simulink model "lyapunov11"  (R2015a)
settings: Solver=ode4  StartTime=0.0  StopTime=15  FixedStep=0.001  RelTol=1e-3
values from neighbouring files (symbols this model uses):
  a = 0.15    [RunLyapunov11.m]    (also in lyapunovInit.m = 0.13)
  kpsi = 10    [RunLyapunov11.m]    (also in lyapunovInit.m)
  kx = 10    [RunLyapunov11.m]    (also in lyapunovInit.m = 25)
  ky = 10    [RunLyapunov11.m]    (also in lyapunovInit.m = 25)
  r = 0.1    [RunLyapunov11.m]    (also in lyapunovInit.m)
  R = 2    [RunLyapunov11.m]    (also in lyapunovInit.m)
  theta0 = pi    (= 3.14159265359)    [RunLyapunov11.m]    (also in lyapunovInit.m)
  wd = 0.5    [RunLyapunov11.m]    (also in lyapunovInit.m)
  x0 = 2.3    [RunLyapunov11.m]    (also in lyapunovInit.m)
  y0 = 0    [RunLyapunov11.m]    (also in lyapunovInit.m)
undefined symbols (not defined in the file or in its folder): lyapu
settings Model: CovModelRefEnable=off  Creator=Subodh  LastModifiedBy=smishra
settings DataIOCC: LimitDataPoints=off  SaveFormat=Dataset
settings HardwareCC: ProdBitPerPointer=64  ProdLargestAtomicFloat=Float  ProdIntDivRoundTo=Zero  ProdEndianess=LittleEndian  ProdHWDeviceType=Specified
settings GRTTargetCC: GeneratePreprocessorConditionals=Use local settings

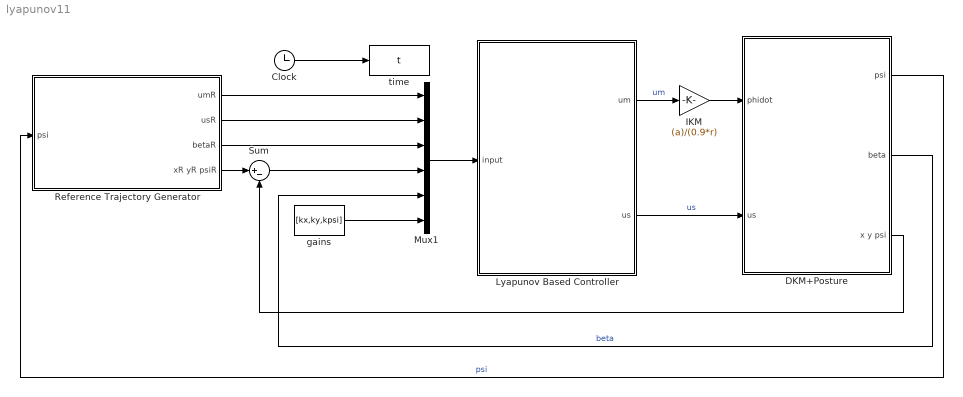
== system lyapunov11 ==
  Clock : Clock
  DKM+Posture : Subsystem
  IKM : Gain  Gain=(a)/(0.9*r)
  Lyapunov Based Controller : Subsystem
  Mux1 : Mux  Inputs=6
  Reference Trajectory Generator : Subsystem
  Sum : Sum  Inputs=|+-
  gains : Constant  Value=[kx,ky,kpsi]
  time : ToWorkspace  VariableName=t  SampleTime=-1
  wires:
  Lyapunov Based Controller/2(us) -> DKM+Posture/2(us)  "us"
  Lyapunov Based Controller/1(um) -> IKM/1  "um"
  IKM/1 -> DKM+Posture/1(phidot)
  DKM+Posture/3(x y psi) -> Sum/2
  Clock/1 -> time/1
  Reference Trajectory Generator/1(umR) -> Mux1/1
  Reference Trajectory Generator/2(usR) -> Mux1/2
  Reference Trajectory Generator/3(betaR) -> Mux1/3
  Reference Trajectory Generator/4(xR yR psiR) -> Sum/1
  Sum/1 -> Mux1/4
  DKM+Posture/2(beta) -> Mux1/5  "beta"
  DKM+Posture/1(psi) -> Reference Trajectory Generator/1(psi)  "psi"
  Mux1/1 -> Lyapunov Based Controller/1(input)
  gains/1 -> Mux1/6

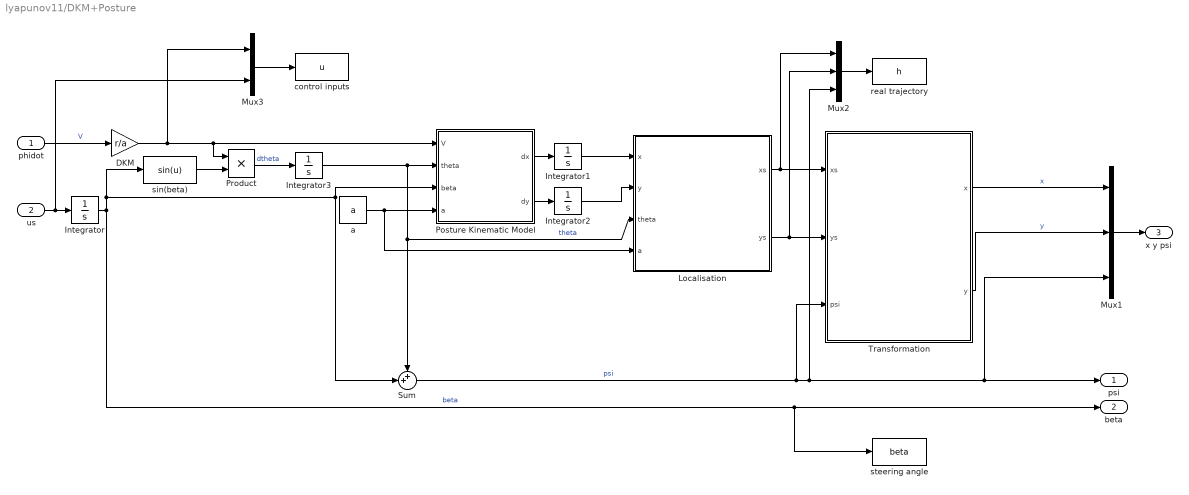
== system lyapunov11/DKM+Posture ==
  phidot : Inport
  us : Inport  Port=2
  DKM : Gain  Gain=r/a
  Integrator : Integrator
  Integrator1 : Integrator  InitialCondition=x0
  Integrator2 : Integrator  InitialCondition=y0
  Integrator3 : Integrator  InitialCondition=theta0
  Localisation : MATLAB Function  TreatAsAtomicUnit=on
  Mux1 : Mux  Inputs=3
  Mux2 : Mux  Inputs=3
  Mux3 : Mux  Inputs=2
  Posture Kinematic Model : MATLAB Function  TreatAsAtomicUnit=on
  Product : Product
  Sum : Sum  Inputs=++|
  Transformation : MATLAB Function  TreatAsAtomicUnit=on
  a : Constant  Value=a
  control inputs : ToWorkspace  VariableName=u  SampleTime=-1
  real trajectory : ToWorkspace  VariableName=h  SampleTime=-1
  sin(beta) : Fcn  Expr=sin(u)
  steering angle : ToWorkspace  VariableName=beta  SampleTime=-1
  psi : Outport
  beta : Outport  Port=2
  x y psi : Outport  Port=3
  wires:
  sin(beta)/1 -> Product/2
  us/1 -> Mux3/2, Integrator/1
  Product/1 -> Integrator3/1  "dtheta"
  Sum/1 -> Transformation/3(psi), Mux2/3, psi/1, Mux1/3  "psi"
  Integrator3/1 -> Sum/1, Localisation/3(theta), Posture Kinematic Model/2(theta)  "theta"
  Posture Kinematic Model/1(dx) -> Integrator1/1
  Posture Kinematic Model/2(dy) -> Integrator2/1
  Integrator/1 -> sin(beta)/1, Posture Kinematic Model/3(beta), Sum/2, steering angle/1, beta/1  "beta"
  Integrator2/1 -> Localisation/2(y)
  Localisation/2(ys) -> Mux2/2, Transformation/2(ys)
  DKM/1 -> Mux3/1, Product/1, Posture Kinematic Model/1(V)
  phidot/1 -> DKM/1  "V"
  Transformation/1(x) -> Mux1/1  "x"
  Transformation/2(y) -> Mux1/2  "y"
  Mux1/1 -> x y psi/1
  a/1 -> Localisation/4(a), Posture Kinematic Model/4(a)
  Integrator1/1 -> Localisation/1(x)
  Localisation/1(xs) -> Mux2/1, Transformation/1(xs)
  Mux2/1 -> real trajectory/1
  Mux3/1 -> control inputs/1

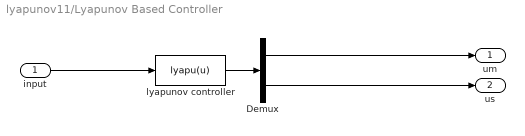
== system lyapunov11/Lyapunov Based Controller ==
  input : Inport
  Demux : Demux  Outputs=2
  lyapunov controller : MATLABFcn  MATLABFcn=lyapu(u)  OutputDimensions=2
  um : Outport
  us : Outport  Port=2
  wires:
  input/1 -> lyapunov controller/1
  Demux/2 -> us/1
  Demux/1 -> um/1
  lyapunov controller/1 -> Demux/1

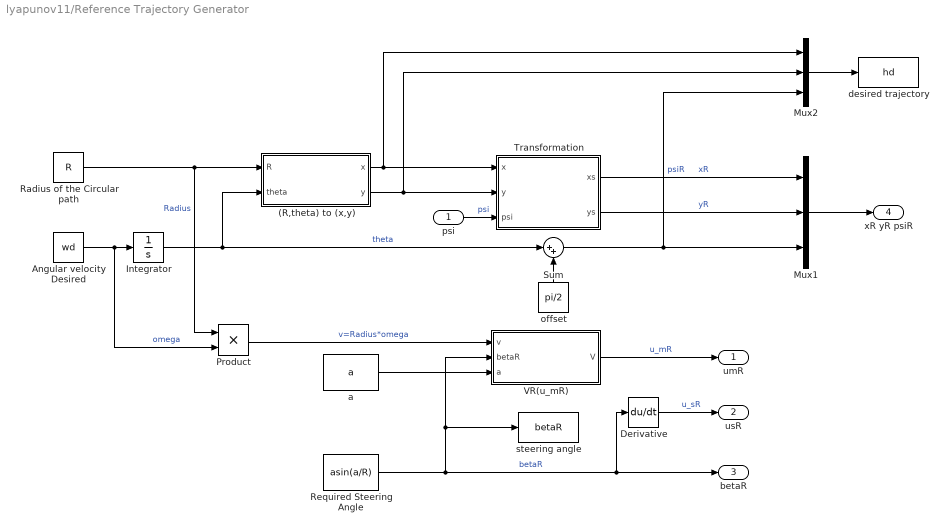
== system lyapunov11/Reference Trajectory Generator ==
  psi : Inport
  (R,theta) to (x,y) : MATLAB Function  TreatAsAtomicUnit=on
  Angular velocity Desired : Constant  Value=wd
  Derivative : Derivative
  Integrator : Integrator
  Mux1 : Mux  Inputs=3
  Mux2 : Mux  Inputs=3
  Product : Product
  Radius of the Circular path : Constant  Value=R
  Required Steering Angle : Constant  Value=asin(a/R)
  Sum : Sum  Inputs=|++
  Transformation : MATLAB Function  TreatAsAtomicUnit=on
  VR(u_mR) : MATLAB Function  TreatAsAtomicUnit=on
  a : Constant  Value=a
  desired trajectory : ToWorkspace  VariableName=hd  SampleTime=-1
  offset : Constant  Value=pi/2
  steering angle : ToWorkspace  VariableName=betaR  SampleTime=-1
  umR : Outport
  usR : Outport  Port=2
  betaR : Outport  Port=3
  xR yR psiR : Outport  Port=4
  wires:
  Radius of the Circular path/1 -> Product/1, (R,theta) to (x,y)/1(R)  "Radius"
  Angular velocity Desired/1 -> Product/2, Integrator/1  "omega"
  VR(u_mR)/1(V) -> umR/1  "u_mR"
  Required Steering Angle/1 -> Derivative/1, betaR/1, steering angle/1, VR(u_mR)/2(betaR)  "betaR"
  Derivative/1 -> usR/1  "u_sR"
  Product/1 -> VR(u_mR)/1(v)  "v=Radius*omega"
  psi/1 -> Transformation/3(psi)  "psi"
  Transformation/1(xs) -> Mux1/1  "xR"
  Transformation/2(ys) -> Mux1/2  "yR"
  (R,theta) to (x,y)/1(x) -> Mux2/1, Transformation/1(x)
  (R,theta) to (x,y)/2(y) -> Mux2/2, Transformation/2(y)
  offset/1 -> Sum/2
  Integrator/1 -> (R,theta) to (x,y)/2(theta), Sum/1  "theta"
  Mux1/1 -> xR yR psiR/1
  a/1 -> VR(u_mR)/3(a)
  Sum/1 -> Mux2/3, Mux1/3  "psiR"
  Mux2/1 -> desired trajectory/1

== matlab function lyapunov11/Reference Trajectory Generator/(R,theta) to (x,y) ==
  data: x output; y output; R input; theta input
function [x,y]= fcn(R,theta)
%#codegen
x=R*cos(theta);
y=R*sin(theta);

== matlab function lyapunov11/Reference Trajectory Generator/Transformation ==
  data: xs output; x input; y input; psi input; ys output
function [xs,ys]= fcn(x,y,psi)
%#codegen
xs=x*cos(psi)+y*sin(psi);
ys=-x*sin(psi)+y*cos(psi);

== matlab function lyapunov11/Reference Trajectory Generator/VR(u_mR) ==
  data: V output; v input; betaR input; a input
function V = fcn(v,betaR,a)
%#codegen
V=v/(a*cos(betaR));

== matlab function lyapunov11/DKM+Posture/Posture Kinematic Model ==
  data: V input; theta input; beta input; dx output; dy output; a input
function [dx,dy] = fcn(V,theta,beta,a)
%#codegen

dx=a*V*cos(theta)*cos(beta);
dy=a*V*sin(theta)*cos(beta);

== matlab function lyapunov11/DKM+Posture/Localisation ==
  data: x input; y input; theta input; xs output; ys output; a input
function [xs,ys] = fcn(x,y,theta,a)
%#codegen

xs=x+a*cos(theta);
ys=y+a*sin(theta);

== matlab function lyapunov11/DKM+Posture/Transformation ==
  data: xs input; ys input; x output; y output; psi input
function [x,y]= fcn(xs,ys,psi)
%#codegen
x=xs*cos(psi)+ys*sin(psi);
y=-xs*sin(psi)+ys*cos(psi);
